simulink model "MOD5UsingJunctions"  (R2020b)
settings: Solver=VariableStepAuto  StartTime=0.0  StopTime=10.0  RelTol=1e-3
settings Model: Creator=BIDITA PAUL  LastModifiedBy=BIDITA PAUL

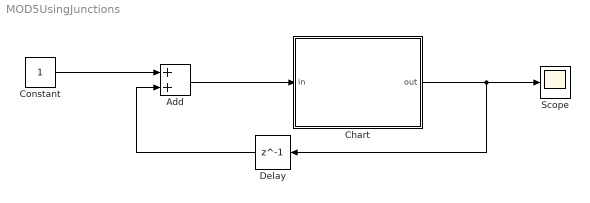
== system MOD5UsingJunctions ==
  Add : Sum
  Chart : Stateflow chart  TreatAsAtomicUnit=on
  Constant : Constant
  Delay : Delay  DelayLength=1
  Scope : Scope
  wires:
  Add/1 -> Chart/1(in)
  Constant/1 -> Add/1
  Chart/1(out) -> Delay/1, Scope/1
  Delay/1 -> Add/2

== stateflow chart MOD5UsingJunctions/Chart ==
  (default) -> (junction 1)
  (junction 1) -> (junction 2) [order 1] : [in<=5]
  (junction 2) -> (junction 3) : {out=in;}
  (junction 1) -> (junction 4) [order 2] : [in>5]
  (junction 3) -> (junction 6)
  (junction 4) -> (junction 5) : {out=0;}
  (junction 5) -> (junction 6)
  data: out output; in input
